simulink model "Acceleration_Model_testing"  (R2020b)
settings: Solver=VariableStepAuto  StartTime=0.0  StopTime=46  MaxStep=0.001  RelTol=1e-3
values from neighbouring files (symbols this model uses):
  Controller_sampleTime = 0.001    [PLC_setup_Rev1_02Mar21.m]    (also in PLC_setup_Rev3.m; PLC_setup_Rev4.m)
undefined symbols (not defined in the file or in its folder): test398_20210427_190936
libraries: simulink x1
settings Model: Creator=JillMacPherson  LastModifiedBy=JillMacPherson

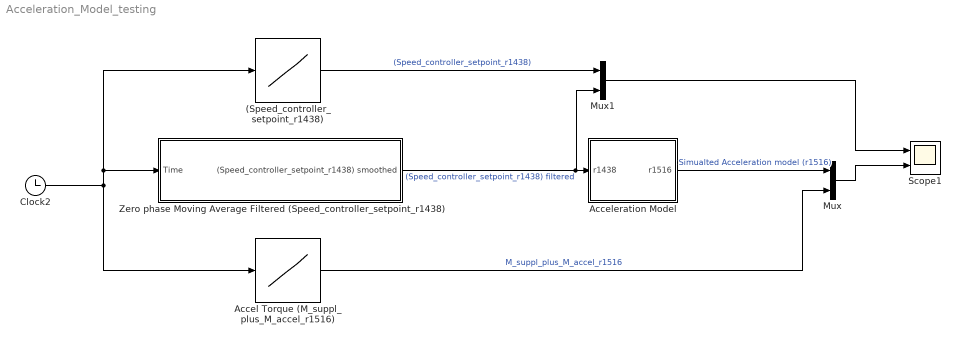
== system Acceleration_Model_testing ==
  (Speed_controller_setpoint_r1438) : Lookup_n-D  NumberOfTableDimensions=1  BreakpointsForDimension1=test398_20210427_190936.fileinfo.Time  Table=test398_20210427_190936.Drive_2.Speed_controller_setpoint_r1438.data  InternalRulePriority=Speed  RndMeth=Simplest  InputSameDT=on
  Accel Torque (M_suppl_plus_M_accel_r1516) : Lookup_n-D  NumberOfTableDimensions=1  BreakpointsForDimension1=test398_20210427_190936.fileinfo.Time  Table=test398_20210427_190936.Drive_2.M_suppl_plus_M_accel_r1516.data  InternalRulePriority=Speed  RndMeth=Simplest  InputSameDT=on
  "Acceleration Model " : Subsystem  TreatAsAtomicUnit=on  SystemSampleTime=0.001
  Clock2 : Clock
  Mux : Mux  Inputs=2
  Mux1 : Mux  Inputs=2
  Scope1 : Scope  NumInputPorts=2
  Zero phase Moving Average Filtered (Speed_controller_setpoint_r1438) : Subsystem  TreatAsAtomicUnit=on  SystemSampleTime=0.001
  wires:
  Clock2/1 -> Zero phase Moving Average Filtered (Speed_controller_setpoint_r1438)/1(Time), (Speed_controller_setpoint_r1438)/1, Accel Torque (M_suppl_plus_M_accel_r1516)/1
  Accel Torque (M_suppl_plus_M_accel_r1516)/1 -> Mux/2  "M_suppl_plus_M_accel_r1516"
  Mux/1 -> Scope1/2
  Mux1/1 -> Scope1/1
  "Acceleration Model "/1(r1516) -> Mux/1  "Simualted Acceleration model (r1516)"
  (Speed_controller_setpoint_r1438)/1 -> Mux1/1  "(Speed_controller_setpoint_r1438)"
  Zero phase Moving Average Filtered (Speed_controller_setpoint_r1438)/1((Speed_controller_setpoint_r1438) smoothed) -> Mux1/2, "Acceleration Model "/1(r1438)  "(Speed_controller_setpoint_r1438) filtered"

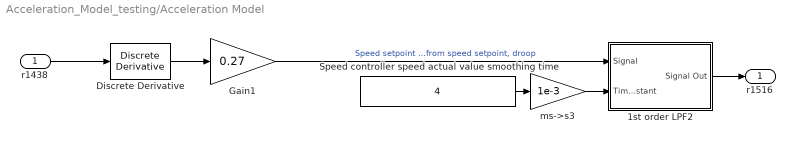
== system Acceleration_Model_testing/Acceleration Model  ==
  r1438 : Inport
  1st order LPF2 : Subsystem  mask{time_constant=0.1, Yo=0}
      mask prompts: time_constant "Time Constant (s)"; Yo "Initial Condition"
  Discrete Derivative : simulink/Discrete/Discrete Derivative  gainval=1.0  ICPrevScaledInput=0.0  OutMin=[]  OutMax=[]  OutDataType=fixdt(1, 16)  OutScaling=2^-10  DoSatur=off
  Gain1 : Gain  Gain=0.27
  Speed controller speed actual value smoothing time : Constant  Value=4
  ms->s3 : Gain  Gain=1e-3
  r1516 : Outport
  wires:
  Discrete Derivative/1 -> Gain1/1
  Speed controller speed actual value smoothing time/1 -> ms->s3/1
  Gain1/1 -> 1st order LPF2/1(Signal)  "Speed setpoint from speed setpoint, droop"
  ms->s3/1 -> 1st order LPF2/2(Time Constant)
  1st order LPF2/1(Signal Out) -> r1516/1
  r1438/1 -> Discrete Derivative/1

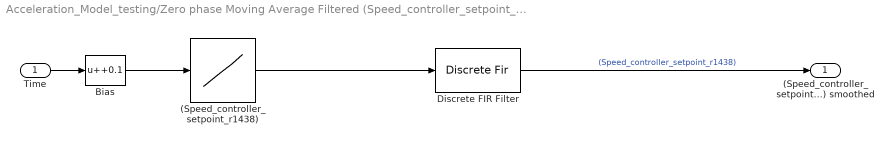
== system Acceleration_Model_testing/Zero phase Moving Average Filtered (Speed_controller_setpoint_r1438) ==
  Time : Inport
  (Speed_controller_setpoint_r1438) : Lookup_n-D  NumberOfTableDimensions=1  BreakpointsForDimension1=test398_20210427_190936.fileinfo.Time  Table=test398_20210427_190936.Drive_2.Speed_controller_setpoint_r1438.data  InternalRulePriority=Speed  RndMeth=Simplest  InputSameDT=on
  Bias : Bias  Bias=+0.1
  Discrete FIR Filter : DiscreteFir  Coefficients=ones(1,200)*0.005
  (Speed_controller_setpoint_r1438) smoothed : Outport
  wires:
  Time/1 -> Bias/1
  Discrete FIR Filter/1 -> (Speed_controller_setpoint_r1438) smoothed/1  "(Speed_controller_setpoint_r1438)"
  (Speed_controller_setpoint_r1438)/1 -> Discrete FIR Filter/1
  Bias/1 -> (Speed_controller_setpoint_r1438)/1

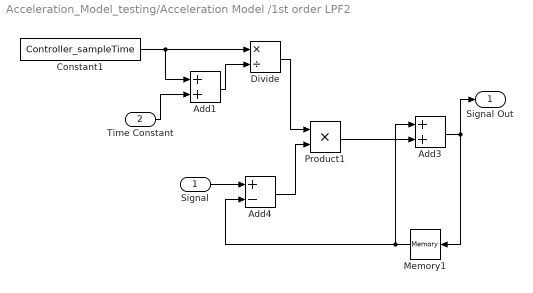
== system Acceleration_Model_testing/Acceleration Model /1st order LPF2 ==
  Signal : Inport
  Time Constant : Inport  Port=2
  Add1 : Sum
  Add3 : Sum
  Add4 : Sum  Inputs=+-
  Constant1 : Constant  Value=Controller_sampleTime
  Divide : Product  Inputs=*/
  Memory1 : Memory  InitialCondition=Yo  InheritSampleTime=on
  Product1 : Product  RndMeth=Zero
  Signal Out : Outport  VectorParamsAs1DForOutWhenUnconnected=off
  wires:
  Signal/1 -> Add4/1
  Constant1/1 -> Divide/1, Add1/1
  Time Constant/1 -> Add1/2
  Add4/1 -> Product1/2
  Memory1/1 -> Add3/1, Add4/2
  Product1/1 -> Add3/2
  Add3/1 -> Signal Out/1, Memory1/1
  Divide/1 -> Product1/1
  Add1/1 -> Divide/2
